simulink model "slider_mode_controller_kalman_filter_sim"  (R2022a)
settings: Solver=VariableStepAuto  StartTime=0.0  StopTime=1000  RelTol=1e-3
undefined symbols (not defined in the file): sim_r
settings Model: Creator=alefr  LastModifiedBy=Alghisi
settings DataIOCC: ReturnWorkspaceOutputs=off
settings DebuggingCC: UnconnectedInputMsg=warning  UnconnectedOutputMsg=warning  UnconnectedLineMsg=warning
settings RTWCC: DLArmComputeVersion=19.05

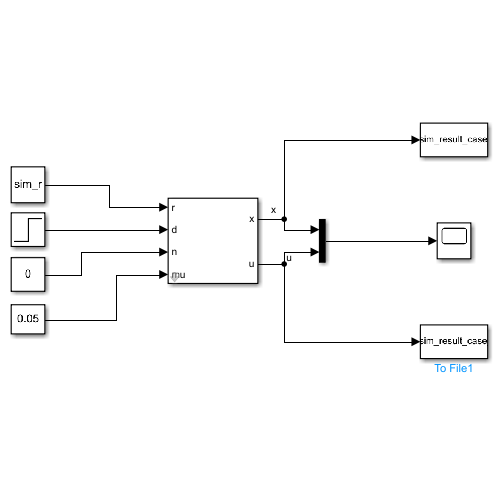
[thumbnail: Simulink's stored preview of the top-level diagram]
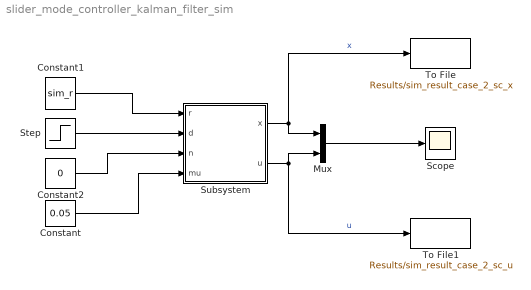
== system slider_mode_controller_kalman_filter_sim ==
  Constant : Constant  Value=0.05
  Constant1 : Constant  Value=sim_r
  Constant2 : Constant  Value=0
  Mux : Mux  Inputs=2
  Scope : Scope
  Step : Step  Time=200  After=0.05  SampleTime=0
  Subsystem : Subsystem  mask{init_state_param=[8;8]}
  To File : ToFile  Filename=Results/sim_result_case_2_sc_x  MatrixName=sim_result_case_2_sc_x  SaveFormat=Timeseries
  To File1 : ToFile  Filename=Results/sim_result_case_2_sc_u  MatrixName=sim_result_case_2_sc_u  SaveFormat=Timeseries
  wires:
  Constant1/1 -> Subsystem/1(r)
  Constant/1 -> Subsystem/4(mu)
  Constant2/1 -> Subsystem/3(n)
  Subsystem/1(x) -> To File/1, Mux/1  "x"
  Subsystem/2(u) -> To File1/1, Mux/2  "u"
  Step/1 -> Subsystem/2(d)
  Mux/1 -> Scope/1

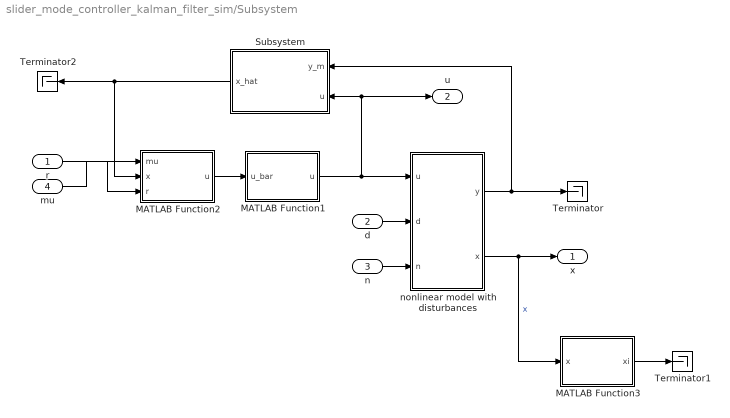
== system slider_mode_controller_kalman_filter_sim/Subsystem ==
  r : Inport
  d : Inport  Port=2
  n : Inport  Port=3
  mu : Inport  Port=4
  MATLAB Function1 : MATLAB Function  TreatAsAtomicUnit=on
  MATLAB Function2 : MATLAB Function  TreatAsAtomicUnit=on
  MATLAB Function3 : MATLAB Function  TreatAsAtomicUnit=on
  Subsystem : Subsystem
  Terminator : Terminator
  Terminator1 : Terminator
  Terminator2 : Terminator
  nonlinear model with disturbances : Subsystem
  x : Outport
  u : Outport  Port=2
  wires:
  MATLAB Function1/1(u) -> u/1, Subsystem/2(u), nonlinear model with disturbances/1(u)
  r/1 -> MATLAB Function2/3(r)
  nonlinear model with disturbances/2(x) -> x/1, MATLAB Function3/1(x)  "x"
  MATLAB Function3/1(xi) -> Terminator1/1
  Subsystem/1(x_hat) -> Terminator2/1, MATLAB Function2/2(x)
  nonlinear model with disturbances/1(y) -> Terminator/1, Subsystem/1(y_m)
  d/1 -> nonlinear model with disturbances/2(d)
  MATLAB Function2/1(u) -> MATLAB Function1/1(u_bar)
  n/1 -> nonlinear model with disturbances/3(n)
  mu/1 -> MATLAB Function2/1(mu)

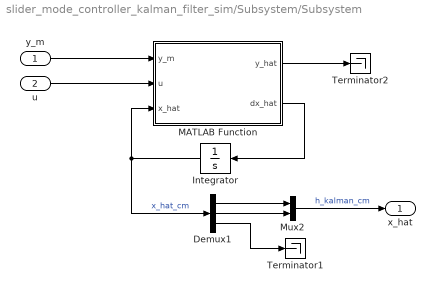
== system slider_mode_controller_kalman_filter_sim/Subsystem/Subsystem ==
  y_m : Inport
  u : Inport  Port=2
  Demux1 : Demux  Outputs=3
  Integrator : Integrator  InitialCondition=[init_state_param;0]
  MATLAB Function : MATLAB Function  TreatAsAtomicUnit=on
  Mux2 : Mux  Inputs=2
  Terminator1 : Terminator
  Terminator2 : Terminator
  x_hat : Outport
  wires:
  Demux1/3 -> Terminator1/1
  Demux1/1 -> Mux2/1
  Demux1/2 -> Mux2/2
  Integrator/1 -> Demux1/1, MATLAB Function/3(x_hat)  "x_hat_cm"
  u/1 -> MATLAB Function/2(u)
  y_m/1 -> MATLAB Function/1(y_m)
  MATLAB Function/1(y_hat) -> Terminator2/1
  MATLAB Function/2(dx_hat) -> Integrator/1
  Mux2/1 -> x_hat/1  "h_kalman_cm"

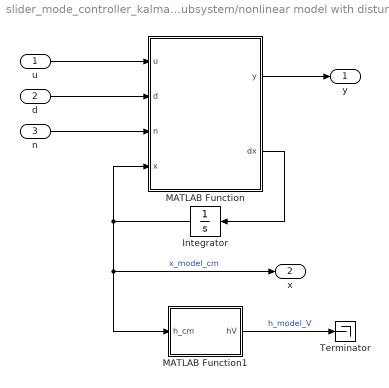
== system slider_mode_controller_kalman_filter_sim/Subsystem/nonlinear model with disturbances ==
  u : Inport
  d : Inport  Port=2
  n : Inport  Port=3
  Integrator : Integrator  InitialCondition=init_state_param
  MATLAB Function : MATLAB Function  TreatAsAtomicUnit=on
  MATLAB Function1 : MATLAB Function  TreatAsAtomicUnit=on
  Terminator : Terminator
  y : Outport
  x : Outport  Port=2
  wires:
  MATLAB Function/1(y) -> y/1
  n/1 -> MATLAB Function/3(n)
  MATLAB Function1/1(hV) -> Terminator/1  "h_model_V"
  d/1 -> MATLAB Function/2(d)
  MATLAB Function/2(dx) -> Integrator/1
  Integrator/1 -> MATLAB Function/4(x), MATLAB Function1/1(h_cm), x/1  "x_model_cm"
  u/1 -> MATLAB Function/1(u)

== matlab function slider_mode_controller_kalman_filter_sim/Subsystem/Subsystem/MATLAB Function ==
  data: y_hat output; y_m input; u input; x_hat input; dx_hat output
function [y_hat,dx_hat]  = kalman_filter(y_m,u,x_hat)

x1_hat = x_hat(1);
x2_hat = x_hat(2);
x3_hat = x_hat(3);

dx_hat = [x1_hat.*(-3.409145021215564e-2)-x2_hat.*4.707003693403074e-1+u.*2.098905560223644e-1+y_m.*6.312683508484582e-1-sqrt(5.0).*sqrt(7.63e+2).*x3_hat.*(4.0./5.5e+1)+9.799223895936307e-1;
    x1_hat.*3.409145021215564e-2-x2_hat.*1.823621215877479e-1+y_m.*1.98849604323964e-1+3.277173484388494e-1;x2_hat.*7.456422751238219e-3-y_m./1.0e+2-1.648066384406454e-2];

y_hat = x2_hat.*7.456422751238219e-1-1.648066384406454;

end

== matlab function slider_mode_controller_kalman_filter_sim/Subsystem/MATLAB Function2 ==
  data: mu input; x input; r input; u output
function u = fcn(mu,x,r)

x1=x(1);
x2=x(2);

u = sqrt(2.9e+1).*sqrt(x1.*5.0+1.6e+1).*(sqrt(2.9e+1).*(sqrt(x1.*5.0+1.6e+1).*7.609042393596842e-2-sqrt(x2.*5.0+1.6e+1).*7.609042393596842e-2).*(2.0./2.9e+1)+sqrt(2.9e+1).*1.0./sqrt(x1.*5.0+1.6e+1).*1.0./sqrt(x2.*5.0+1.6e+1).*(x1.*2.7795e+4+8.8944e+4).*6.020670028073036e-7).*(-3.469556172037643e+1)-sqrt(2.9e+1).*mu.*sqrt(x1.*5.0+1.6e+1).*min([1.0,max([-1.0,-r+x2.*7.456422751238219e-1+sqrt(x1.*1.962e+3+6.2784e+3).*9.602968694776494e-3-sqrt(x2.*1.962e+3+6.2784e+3).*9.602968694776494e-3-1.648066384406454],[],2,'omitnan')],[],2,'omitnan').*3.469556172037643e+1;
end

== matlab function slider_mode_controller_kalman_filter_sim/Subsystem/MATLAB Function1 ==
  data: u_bar input; u output
function u = pm1(u_bar)

u = u_bar.*3.277899884284337e-1-u_bar.^2.*9.88758313621772e-3+u_bar.^3.*1.567756031883916e-4-2.914041336753123;

end

== matlab function slider_mode_controller_kalman_filter_sim/Subsystem/MATLAB Function3 ==
  data: x input; xi output
function xi = T(x)

x1 = x(1);
x2 = x(2);

xi = [x2.*7.456422751238219e-1-1.648066384406454;sqrt(x1.*1.962e+3+6.2784e+3).*3.841187477910597e-3-sqrt(x2.*1.962e+3+6.2784e+3).*3.841187477910597e-3];

end

== matlab function slider_mode_controller_kalman_filter_sim/Subsystem/nonlinear model with disturbances/MATLAB Function ==
  data: y output; u input; dx output; d input; n input; x input
function [y,dx] = nonlinear_model(u,d,n,x)

x1 = x(1);
x2 = x(2);

y = x2.*7.456422751238219e-1 + n -1.648066384406454;

dx = [+u.*2.81859116712929e-1-(d.*sqrt(x1.*1.962e+3+6.2784e+3))./3.3e+1-sqrt(x1.*1.962e+3+6.2784e+3).*5.151515151515152e-3-u.^2.*2.476601319356692e-2+u.^3.*8.808489605974731e-4+3.751072019731428e-1;sqrt(x1.*1.962e+3+6.2784e+3).*5.151515151515152e-3-sqrt(x2.*1.962e+3+6.2784e+3).*5.151515151515152e-3];

end

== matlab function slider_mode_controller_kalman_filter_sim/Subsystem/nonlinear model with disturbances/MATLAB Function1 ==
  data: h_cm input; hV output
function hV = g(h_cm)

hV = h_cm*7.456422751238219e-1 - 1.648066384406454;
